simulink model "TEST_half_bridge"  (R2023a)
settings: Solver=FixedStepAuto  StartTime=0.0  StopTime=0.1  FixedStep=SampleTime  MaxStep=1e-4  RelTol=1e-8
InitFcn:
  | F = 10;
  | Fc = 10*F;
values from neighbouring files (symbols this model uses):
  L_load = 10e-3    (= 0.01)    [preload.m]
  R_load = 1e-3    (= 0.001)    [preload.m]
  SampleTime = 10e-8    (= 1e-07)    [preload.m]
  Sequence_amplitude = 1    [preload.m]
  Sequence_frequency = fs    (= 2550)    [preload.m]
  V_control_amplitude = ma    (= 0.85)    [preload.m]
  V_control_frequency = V_grid_frequency    (= 314.159265359)    [preload.m]
  V_grid_amplitude = sqrt(2)*240    [preload.m]
  V_grid_frequency = 2*pi*50    (= 314.159265359)    [preload.m]
  Vdc = 752    [preload.m]
undefined symbols (not defined in the file or in its folder): Va_grid_amplitude, Va_grid_frequency, Va_grid_phase
libraries: spsGroundLib x4, spsVoltageMeasurementLib x3, spsCurrentMeasurementLib x2, spsMosfetLib x2, spsDCVoltageSourceLib x2, spsControlledVoltageSourceLib x1, simulink x1, spsSeriesRLCBranchLib x1, spspowerguiLib x1
settings Model: Creator=ADMIN  LastModifiedBy=ADMIN
settings DataIOCC: ReturnWorkspaceOutputsName=out_half

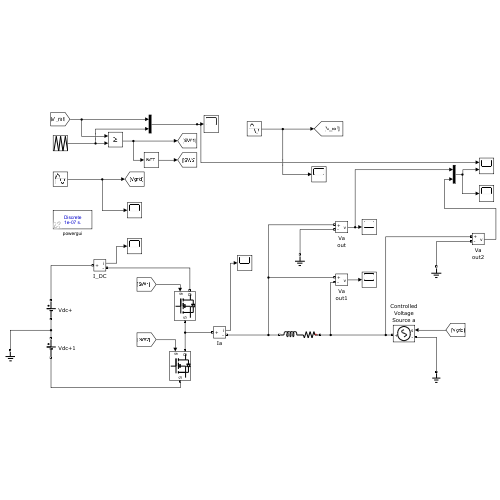
[thumbnail: Simulink's stored preview of the top-level diagram]
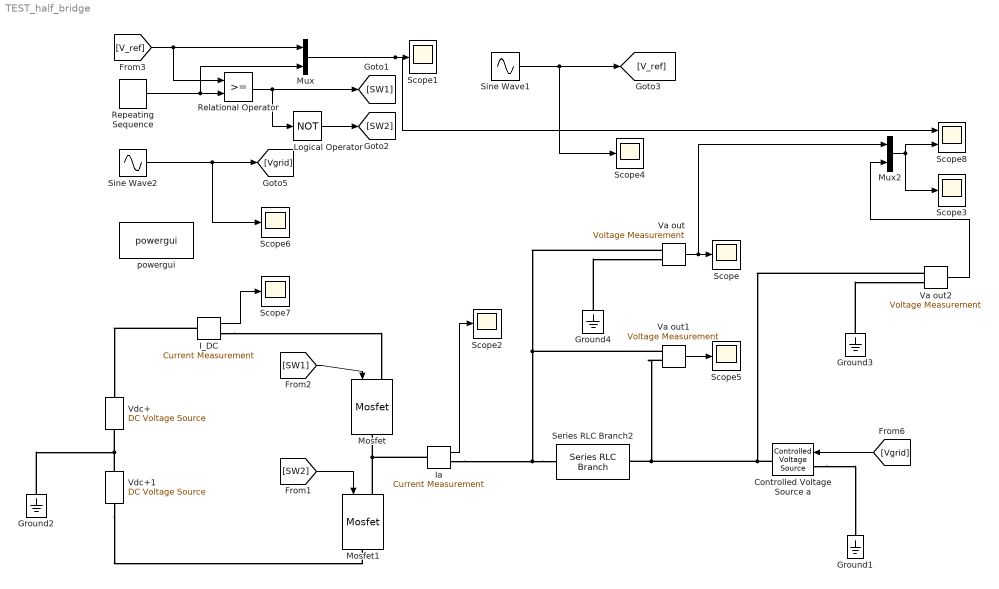
== system TEST_half_bridge ==
  Controlled Voltage Source a : spsControlledVoltageSourceLib/Controlled Voltage Source  Initialize=off  Source_Type=AC  Amplitude=Va_grid_amplitude  Phase=Va_grid_phase  Frequency=Va_grid_frequency  Measurements=None
  Ground{1..4} (4 alike) : spsGroundLib/Ground  LConnTagsString=a
  I_DC : spsCurrentMeasurementLib/Current Measurement  PhasorSimulation=off  OutputType=Complex  PSBequivalent=0
  Ia : spsCurrentMeasurementLib/Current Measurement  PhasorSimulation=off  OutputType=Complex  PSBequivalent=0
  Logical Operator : Logic  Operator=NOT  AllPortsSameDT=off  OutDataTypeStr=boolean
  Mosfet : spsMosfetLib/Mosfet  Ron=0.1  Lon=0  Rd=0.01  Vfd=0  IC=0  Rs=1e5  Cs=inf  Measurements=off
  Mosfet1 : spsMosfetLib/Mosfet  Ron=0.1  Lon=0  Rd=0.01  Vfd=0  IC=0  Rs=1e5  Cs=inf  Measurements=off
  Mux : Mux  Inputs=2
  Mux2 : Mux  Inputs=2
  Relational Operator : RelationalOperator  OutDataTypeStr=boolean  RndMeth=Simplest  InputSameDT=off
  Repeating Sequence : simulink/Sources/Repeating Sequence  rep_seq_t=[0 1 2]*[1/Sequence_frequency]  rep_seq_y=[-Sequence_amplitude Sequence_amplitude -Sequence_amplitude]
  Scope{,1..7} (8 alike) : Scope
  Scope8 : Scope  NumInputPorts=2
  Series RLC Branch2 : spsSeriesRLCBranchLib/Series RLC Branch  LConnTagsString=__new0  RConnTagsString=__new0  BranchType=RL  Resistance=R_load  Inductance=L_load  SetiL0=off  InitialCurrent=0  Capacitance=1e-6  Setx0=off  InitialVoltage=0  Measurements=None
  Sine Wave1 : Sin  Amplitude=V_control_amplitude  Frequency=V_control_frequency  SampleTime=0
  Sine Wave2 : Sin  Amplitude=V_grid_amplitude  Frequency=V_grid_frequency  SampleTime=0
  Va out : spsVoltageMeasurementLib/Voltage Measurement  PhasorSimulation=off  OutputType=Complex  PSBequivalent=0
  Va out1 : spsVoltageMeasurementLib/Voltage Measurement  PhasorSimulation=off  OutputType=Complex  PSBequivalent=0
  Va out2 : spsVoltageMeasurementLib/Voltage Measurement  PhasorSimulation=off  OutputType=Complex  PSBequivalent=0
  Vdc+ : spsDCVoltageSourceLib/DC Voltage Source  Amplitude=Vdc/2  Measurements=None
  Vdc+1 : spsDCVoltageSourceLib/DC Voltage Source  Amplitude=Vdc/2  Measurements=None
  powergui : spspowerguiLib/powergui  Priority=1  SimulationMode=Discrete  SampleTime=SampleTime  frequency=60  Iterations=50  frequencyindice=0  Pbase=100e6  ErrMax=1e-4  UnitsV=kV  UnitsW=MW  buscounter=0  FunctionMessages=off  echomessages=off  EnableUseOfTLC=off  CurrentSourceSwitches=off  DisableSnubberDevices=off  DisableRonSwitches=off  DisableVfSwitches=off  DisplayEquations=off  AutomaticDiscreteSolvers=off  SolverType=Tustin/Backward Euler (TBE)  Interpol=off  ExternalGateDelay=off  methode=off  Ts=100  x0status=blocks  SPID=on  SwTol=0  HookPort=off  NonlinearTolerance=1e-4  nMaxIteration=100  ContinueOnMaxIteration=off  RestoreLinks=warning  ResistiveCurrentMeasurement=off  Frange=[0:2:500]  Ylog=off  Xlog=on  ShowGrid=off  save=off  variable=ZData  structure=0  ZoomFFT=off  StartTime=0.0  cycles=1  DisplayStyle=1  fundamental=60  FreqAxis=off  MaxFrequency=1000  frequencyindicesteady=1  RmsSteady=1  display=off
  wires:
  Repeating Sequence/1 -> Mux/2, Relational Operator/2
  Relational Operator/1 -> [SW1], Logical Operator/1
  Logical Operator/1 -> [SW2]
  [SW1] -> Mosfet/1
  [SW2] -> Mosfet1/1
  Va out1/1 -> Scope5/1
  Va out/1 -> Mux2/1, Scope/1
  [Vgrid] -> Controlled Voltage Source a/1
  Ia/1 -> Scope2/1
  Sine Wave2/1 -> Scope6/1, [Vgrid]
  Mux/1 -> Scope8/1, Scope1/1
  Sine Wave1/1 -> Scope4/1, [V_ref]
  [V_ref] -> Relational Operator/1, Mux/1
  I_DC/1 -> Scope7/1
  Va out2/1 -> Mux2/2
  Mux2/1 -> Scope3/1, Scope8/2
  connections:
  Mosfet1/LConn1 -- Ia/LConn1 -- Mosfet/RConn1
  Vdc+1/LConn1 -- Mosfet1/RConn1
  Vdc+1/RConn1 -- Ground2/LConn1 -- Vdc+/LConn1
  Series RLC Branch2/LConn1 -- Va out2/LConn1 -- Controlled Voltage Source a/RConn1 -- Va out1/LConn2
  Series RLC Branch2/RConn1 -- Ia/RConn1 -- Va out1/LConn1 -- Va out/LConn1
  Ground4/LConn1 -- Va out/LConn2
  Controlled Voltage Source a/LConn1 -- Ground1/LConn1
  I_DC/LConn1 -- Vdc+/RConn1
  I_DC/RConn1 -- Mosfet/LConn1
  Ground3/LConn1 -- Va out2/LConn2
